simulink model "cvoo_g19_ponto4"  (R2021a)
settings: Solver=VariableStepAuto  StartTime=0.0  StopTime=100  RelTol=1e-3
values from neighbouring files (symbols this model uses):
  b_h_pt = [ ... (first row only)    [Ponto3.m]    (also in Ponto4.m; Ponto5.m)
  c_h_pt = eye(size(a_h_pt))    [Ponto3.m]    (also in Ponto4.m; Ponto5.m)
  conv_max = 5    [Ponto4.m]    (also in Ponto5.m)
  conv_min = 0    [Ponto4.m]    (also in Ponto5.m)
  conv_rms = 1.5*conv_res    (= 0.0018310546875)    [Ponto4.m]    (also in Ponto5.m)
  d_h_pt = zeros(size(b_h_pt))    [Ponto3.m]    (also in Ponto4.m; Ponto5.m)
  deg = pi/180    (= 0.0174532925199)    [Ponto2.m]    (also in Ponto3.m; Ponto4.m; Ponto5.m)
  f_amost = 100    [Ponto4.m]    (also in Ponto5.m)
  fat_conv_ra = 1/3    (= 0.333333333333)    [Ponto4.m]    (also in Ponto5.m)
  G_ra = 10e-3/ft    (= 0.0328083989501)    [Ponto4.m]    (also in Ponto5.m)
  G_sensq = (V_max_sensq-V_min_sensq)/(q_max_sensq-q_min_sensq)    (= 0.006)    [Ponto4.m]    (also in Ponto5.m)
  Gp_din = (v_pdin_max-v_pdin_min)/(pdin_max-pdin_min)    (= 0.00125)    [Ponto4.m]    (also in Ponto5.m)
  h_pt_ref = -1    [Ponto3.m]    (also in Ponto4.m; Ponto5.m = 0)
  h_ra_max = 1500*ft    (= 457.2)    [Ponto4.m]    (also in Ponto5.m)
  h_ra_min = 0    [Ponto4.m]    (also in Ponto5.m)
  K_lqr = lqr(a_h_pt_int, b_h_pt_int, Q, R)    [Ponto3.m]    (also in Ponto4.m; Ponto5.m)
  offset_alt = 150    [Ponto4.m]    (also in Ponto5.m = 0)
  offset_pdin = 2.5    [Ponto4.m]    (also in Ponto5.m)
  Offset_ra = 2.5    [Ponto4.m]    (also in Ponto5.m = 0)
  Offset_sensq = 2.5    [Ponto4.m]    (also in Ponto5.m)
  p_din_tau = 0.01    [Ponto4.m]    (also in Ponto5.m)
  pdin_max = 2e3    (= 2000)    [Ponto4.m]    (also in Ponto5.m)
  pdin_min = -2e3    (= -2000)    [Ponto4.m]    (also in Ponto5.m)
  q_max_sensq = 300    [Ponto4.m]    (also in Ponto5.m)
  q_min_sensq = -300    [Ponto4.m]    (also in Ponto5.m)
  ra_rms = 0.015    [Ponto4.m]    (also in Ponto5.m)
  rad = 180/pi    (= 57.2957795131)    [Ponto2.m]    (also in Ponto3.m; Ponto4.m; Ponto5.m)
  rho0 = 1.225    [Ponto4.m]    (also in Ponto5.m)
  rms_sensq = 4.4    [Ponto4.m]    (also in Ponto5.m)
  tau = 0.1    [Ponto4.m]    (also in Ponto5.m)
  u_ref = 0.4    [Ponto3.m]    (also in Ponto4.m; Ponto5.m = 0)
  vel_max_at = 60    [Ponto4.m]    (also in Ponto5.m)
  x0 = [0 0 0 0]    [Ponto3.m]    (also in Ponto4.m; Ponto5.m)
  x0_e = [0 0 0 0 0]    [Ponto4.m]    (also in Ponto5.m = [0 0 0 0 cond_ini.h0+h_solo_0])
undefined symbols (not defined in the file or in its folder): a_h_pt, ae, be, ce, cond_ini, de, max_deflec
libraries: simulink x5
settings Model: Creator=josem  LastModifiedBy=thomasmchilds
settings SolverCC: AlgebraicLoopSolver=TrustRegion
settings DebuggingCC: SFMachineParentedDataDiag=warning

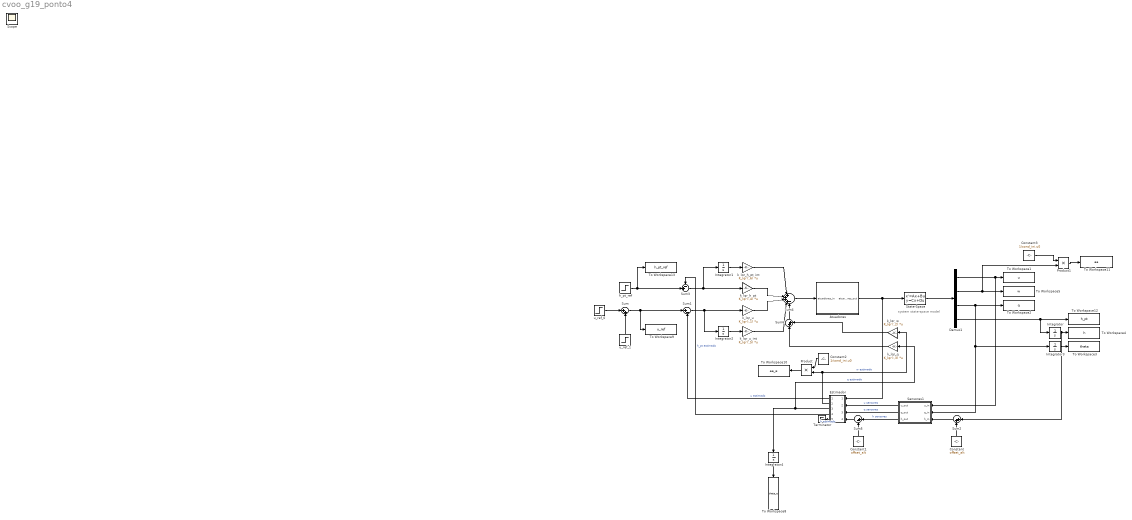
== system cvoo_g19_ponto4 ==
  note: system state-space model
  Atuadores : Subsystem
  Constant : Constant  Value=offset_alt
  Constant1 : Constant  Value=offset_alt
  Constant2 : Constant  Value=1/cond_ini.u0
  Constant3 : Constant  Value=1/cond_ini.u0
  Demux1 : Demux
  Estimador : Subsystem
  Integrator : Integrator
  Integrator1 : Integrator
  Integrator2 : Integrator
  Integrator3 : Integrator  InitialCondition=cond_ini.tt0
  Integrator4 : Integrator  InitialCondition=cond_ini.tt0
  Product : Product
  Product1 : Product
  Sensores1 : Subsystem
  State-Space : StateSpace  A=a_h_pt  B=b_h_pt  C=c_h_pt  D=d_h_pt  InitialCondition=x0
  Sum : Sum  Inputs=|++
  Sum1 : Sum  Inputs=|+-
  Sum2 : Sum  Inputs=|++
  Sum3 : Sum  Inputs=-+|
  Sum4 : Sum  Inputs=|++++-
  Sum5 : Sum  Inputs=|+-
  Sum6 : Sum  Inputs=|++
  Terminator : Terminator
  To Workspace1 : ToWorkspace  VariableName=u  SampleTime=-1
  To Workspace10 : ToWorkspace  VariableName=aa_e  SampleTime=-1
  To Workspace11 : ToWorkspace  VariableName=aa  SampleTime=-1
  To Workspace12 : ToWorkspace  VariableName=h_pt  SampleTime=-1
  To Workspace13 : ToWorkspace  VariableName=h_pt_ref  SampleTime=-1
  To Workspace2 : ToWorkspace  VariableName=q  SampleTime=-1
  To Workspace3 : ToWorkspace  VariableName=theta  SampleTime=-1
  To Workspace4 : ToWorkspace  VariableName=h  SampleTime=-1
  To Workspace5 : ToWorkspace  VariableName=w  SampleTime=-1
  To Workspace8 : ToWorkspace  VariableName=theta_e  SampleTime=-1
  To Workspace9 : ToWorkspace  VariableName=u_ref  SampleTime=-1
  h_pt_ref : Step  Time=50  After=h_pt_ref  SampleTime=0  VectorParams1D=off
  k_lqr_h_pt : Gain  Gain=K_lqr(:,4)  Multiplication=Matrix(K*u)
  k_lqr_h_pt_int : Gain  Gain=K_lqr(:,6)  Multiplication=Matrix(K*u)
  k_lqr_q : Gain  Gain=K_lqr(:,3)  Multiplication=Matrix(K*u)
  k_lqr_u : Gain  Gain=K_lqr(:,1)  Multiplication=Matrix(K*u)
  k_lqr_u_int : Gain  Gain=K_lqr(:,5)  Multiplication=Matrix(K*u)
  k_lqr_w : Gain  Gain=K_lqr(:,2)  Multiplication=Matrix(K*u)
  u_ref_0 : Step  Time=10  After=u_ref  SampleTime=0  VectorParams1D=off
  u_ref_1 : Step  Time=30  After=-u_ref  SampleTime=0
  Scope : Scope
  wires:
  h_pt_ref/1 -> Sum3/2, To Workspace13/1
  u_ref_0/1 -> Sum/1
  Integrator1/1 -> k_lqr_h_pt_int/1
  u_ref_1/1 -> Sum/2
  State-Space/1 -> Demux1/1
  k_lqr_u_int/1 -> Sum4/4
  Sum/1 -> To Workspace9/1, Sum1/1
  Sum1/1 -> Integrator2/1, k_lqr_u/1
  Demux1/3 -> To Workspace2/1, Sensores1/2(q_in), Integrator3/1
  Sum6/1 -> Sum4/5
  k_lqr_h_pt/1 -> Sum4/2
  Demux1/2 -> To Workspace5/1, Product1/2
  k_lqr_u/1 -> Sum4/3
  k_lqr_q/1 -> Sum6/1
  k_lqr_w/1 -> Sum6/2
  Sum4/1 -> Atuadores/1(atuadores_in)
  Demux1/4 -> Integrator/1, To Workspace12/1
  Atuadores/1(atuadores_out) -> State-Space/1, Estimador/1(In1)
  Sum3/1 -> Integrator1/1, k_lqr_h_pt/1
  Demux1/1 -> Sensores1/1(u_in), To Workspace1/1
  Integrator3/1 -> To Workspace3/1
  Integrator2/1 -> k_lqr_u_int/1
  Integrator/1 -> Sum2/1, To Workspace4/1
  k_lqr_h_pt_int/1 -> Sum4/1
  Sensores1/3(h_out) -> Sum5/1  "h sensores"
  Sensores1/2(q_out) -> Estimador/3(q_out)  "q sensores"
  Sum2/1 -> Sensores1/3(h_in)
  Constant/1 -> Sum2/2
  Constant1/1 -> Sum5/2
  Sum5/1 -> Estimador/4(h_out)
  Sensores1/1(u_out) -> Estimador/2(u_out)  "u sensores"
  Estimador/1(Out4) -> Sum1/2  "u estimado"
  Estimador/2(Out2) -> k_lqr_w/1, Product/2  "w estimado"
  Estimador/3(Out3) -> Integrator4/1, k_lqr_q/1  "q estimado"
  Estimador/4(Out1) -> Sum3/1  "h_pt estimado"
  Estimador/5(Out5) -> Terminator/1  "h estimado"
  Integrator4/1 -> To Workspace8/1
  Product/1 -> To Workspace10/1
  Constant2/1 -> Product/1
  Constant3/1 -> Product1/1
  Product1/1 -> To Workspace11/1

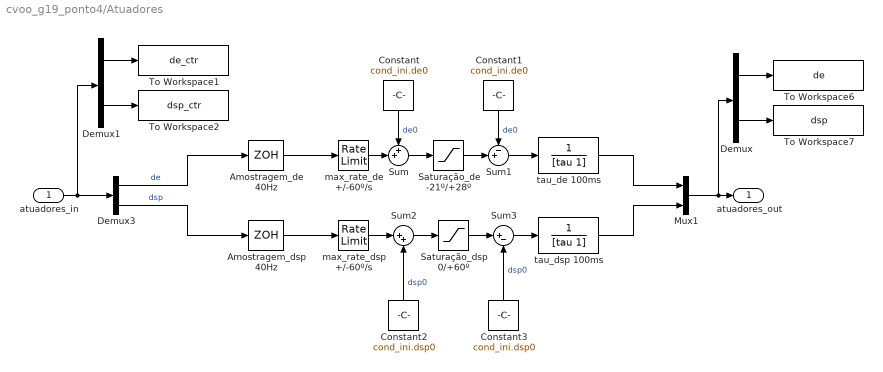
== system cvoo_g19_ponto4/Atuadores ==
  atuadores_in : Inport
  " max_rate_de +/-60º/s" : RateLimiter  RisingSlewLimit=vel_max_at*deg  FallingSlewLimit=-vel_max_at*deg  SampleTimeMode=inherited
  " max_rate_dsp +/-60º/s" : RateLimiter  RisingSlewLimit=vel_max_at*deg  FallingSlewLimit=-vel_max_at*deg  SampleTimeMode=inherited
  Amostragem_de 40Hz : ZeroOrderHold  SampleTime=1/f_amost
  Amostragem_dsp 40Hz : ZeroOrderHold  SampleTime=1/f_amost
  Constant : Constant  Value=cond_ini.de0
  Constant1 : Constant  Value=cond_ini.de0
  Constant2 : Constant  Value=cond_ini.dsp0
  Constant3 : Constant  Value=cond_ini.dsp0
  Demux : Demux  Outputs=2
  Demux1 : Demux  Outputs=2
  Demux3 : Demux  Outputs=2
  Mux1 : Mux  Inputs=2
  Saturação_de -21º/+28º : Saturate  UpperLimit=max_deflec.demax  LowerLimit=max_deflec.demin
  Saturação_dsp 0/+60º : Saturate  UpperLimit=max_deflec.spmax  LowerLimit=0
  Sum : Sum  Inputs=++|
  Sum1 : Sum  Inputs=-+|
  Sum2 : Sum  Inputs=|++
  Sum3 : Sum  Inputs=|+-
  To Workspace1 : ToWorkspace  VariableName=de_ctr  SaveFormat=Structure With Time  SampleTime=-1
  To Workspace2 : ToWorkspace  VariableName=dsp_ctr  SaveFormat=Structure With Time  SampleTime=-1
  To Workspace6 : ToWorkspace  VariableName=de  SaveFormat=Structure With Time  SampleTime=-1
  To Workspace7 : ToWorkspace  VariableName=dsp  SaveFormat=Structure With Time  SampleTime=-1
  tau_de 100ms : TransferFcn  Denominator=[tau 1]
  tau_dsp 100ms : TransferFcn  Denominator=[tau 1]
  atuadores_out : Outport
  wires:
  Mux1/1 -> Demux/1, atuadores_out/1
  atuadores_in/1 -> Demux1/1, Demux3/1
  Demux3/1 -> Amostragem_de 40Hz/1  "de"
  Demux3/2 -> Amostragem_dsp 40Hz/1  "dsp"
  tau_dsp 100ms/1 -> Mux1/2
  tau_de 100ms/1 -> Mux1/1
  Amostragem_dsp 40Hz/1 -> " max_rate_dsp +/-60º/s"/1
  Amostragem_de 40Hz/1 -> " max_rate_de +/-60º/s"/1
  " max_rate_de +/-60º/s"/1 -> Sum/2
  Sum/1 -> Saturação_de -21º/+28º/1
  Constant/1 -> Sum/1  "de0"
  Saturação_de -21º/+28º/1 -> Sum1/2
  Sum1/1 -> tau_de 100ms/1
  Constant1/1 -> Sum1/1  "de0"
  " max_rate_dsp +/-60º/s"/1 -> Sum2/1
  Sum2/1 -> Saturação_dsp 0/+60º/1
  Constant2/1 -> Sum2/2  "dsp0"
  Constant3/1 -> Sum3/2  "dsp0"
  Saturação_dsp 0/+60º/1 -> Sum3/1
  Sum3/1 -> tau_dsp 100ms/1
  Demux/1 -> To Workspace6/1
  Demux/2 -> To Workspace7/1
  Demux1/2 -> To Workspace2/1
  Demux1/1 -> To Workspace1/1

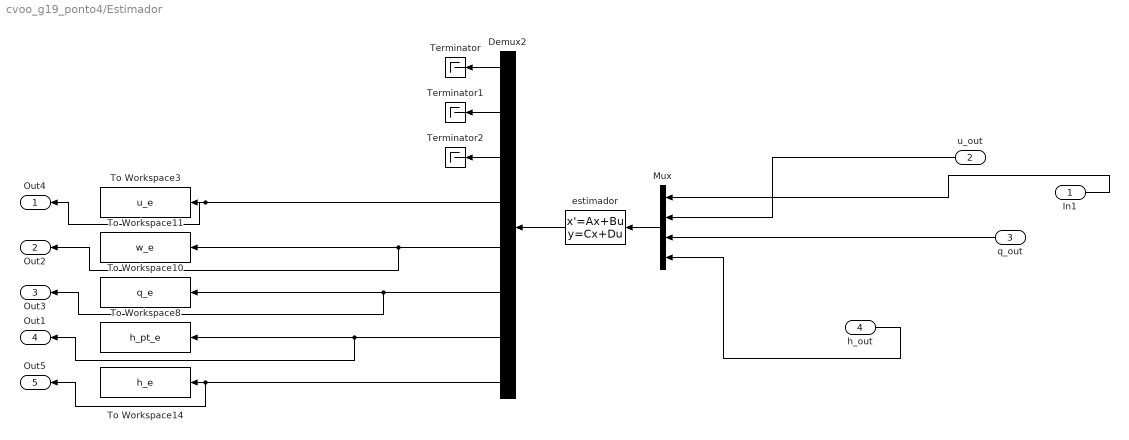
== system cvoo_g19_ponto4/Estimador ==
  In1 : Inport
  u_out : Inport  Port=2
  q_out : Inport  Port=3
  h_out : Inport  Port=4
  Demux2 : Demux  Outputs=8
  Mux : Mux
  Terminator : Terminator
  Terminator1 : Terminator
  Terminator2 : Terminator
  To Workspace10 : ToWorkspace  VariableName=q_e  SampleTime=-1
  To Workspace11 : ToWorkspace  VariableName=w_e  SampleTime=-1
  To Workspace14 : ToWorkspace  VariableName=h_e  SampleTime=-1
  To Workspace3 : ToWorkspace  VariableName=u_e  SampleTime=-1
  To Workspace8 : ToWorkspace  VariableName=h_pt_e  SampleTime=-1
  estimador : StateSpace  A=ae  B=be  C=ce  D=de  InitialCondition=x0_e
  Out4 : Outport
  Out2 : Outport  Port=2
  Out3 : Outport  Port=3
  Out1 : Outport  Port=4
  Out5 : Outport  Port=5
  wires:
  Demux2/2 -> Terminator1/1
  estimador/1 -> Demux2/1
  Demux2/5 -> Out2/1, To Workspace11/1
  Demux2/7 -> Out1/1, To Workspace8/1
  Demux2/8 -> Out5/1, To Workspace14/1
  Demux2/1 -> Terminator/1
  Demux2/4 -> Out4/1, To Workspace3/1
  Demux2/3 -> Terminator2/1
  Mux/1 -> estimador/1
  Demux2/6 -> Out3/1, To Workspace10/1
  In1/1 -> Mux/1
  q_out/1 -> Mux/3
  u_out/1 -> Mux/2
  h_out/1 -> Mux/4

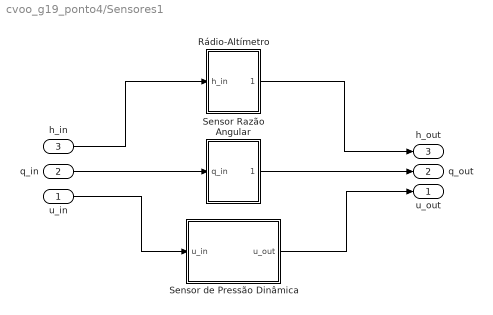
== system cvoo_g19_ponto4/Sensores1 ==
  u_in : Inport
  q_in : Inport  Port=2
  h_in : Inport  Port=3
  Rádio-Altímetro : Subsystem
  Sensor Razão Angular : Subsystem
  Sensor de Pressão Dinâmica : Subsystem
  u_out : Outport
  q_out : Outport  Port=2
  h_out : Outport  Port=3
  wires:
  Sensor Razão Angular/1(q_out) -> q_out/1
  u_in/1 -> Sensor de Pressão Dinâmica/1(u_in)
  Sensor de Pressão Dinâmica/1(u_out) -> u_out/1
  q_in/1 -> Sensor Razão Angular/1(q_in)
  h_in/1 -> Rádio-Altímetro/1(h_in)
  Rádio-Altímetro/1(h_out) -> h_out/1

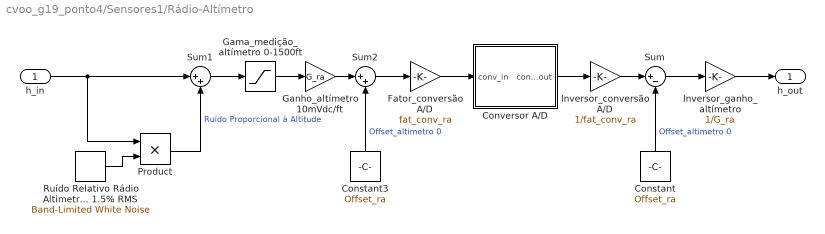
== system cvoo_g19_ponto4/Sensores1/Rádio-Altímetro ==
  h_in : Inport
  Constant : Constant  Value=Offset_ra
  Constant3 : Constant  Value=Offset_ra
  Conversor A/D : Subsystem
  Fator_conversão A/D : Gain  Gain=fat_conv_ra
  Gama_medição_altímetro 0-1500ft : Saturate  UpperLimit=h_ra_max  LowerLimit=h_ra_min
  Ganho_altímetro 10mVdc/ft : Gain  Gain=G_ra
  Inversor_conversão A/D : Gain  Gain=1/fat_conv_ra
  Inversor_ganho_altímetro : Gain  Gain=1/G_ra
  Product : Product
  Ruído Relativo Rádio Altimetro 1.5% RMS : simulink/Sources/Band-Limited White Noise  Cov=[ra_rms^2/f_amost]  Ts=1/f_amost  seed=[23341]
  Sum : Sum  Inputs=|+-
  Sum1 : Sum  Inputs=|++
  Sum2 : Sum  Inputs=|++
  h_out : Outport
  wires:
  Sum/1 -> Inversor_ganho_altímetro/1
  Constant/1 -> Sum/2  "Offset_altimetro 0"
  Sum2/1 -> Fator_conversão A/D/1
  Fator_conversão A/D/1 -> Conversor A/D/1(conv_in)
  Inversor_conversão A/D/1 -> Sum/1
  Conversor A/D/1(conv_out) -> Inversor_conversão A/D/1
  Inversor_ganho_altímetro/1 -> h_out/1
  h_in/1 -> Product/1, Sum1/1
  Sum1/1 -> Gama_medição_altímetro 0-1500ft/1
  Ganho_altímetro 10mVdc/ft/1 -> Sum2/1
  Gama_medição_altímetro 0-1500ft/1 -> Ganho_altímetro 10mVdc/ft/1
  Constant3/1 -> Sum2/2  "Offset_altimetro 0"
  Ruído Relativo Rádio Altimetro 1.5% RMS/1 -> Product/2
  Product/1 -> Sum1/2  "Ruído Proporcional à Altitude"

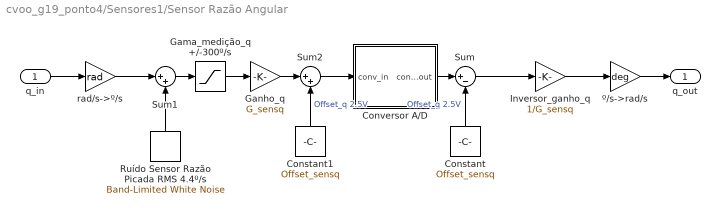
== system cvoo_g19_ponto4/Sensores1/Sensor Razão Angular ==
  q_in : Inport
  Constant : Constant  Value=Offset_sensq
  Constant1 : Constant  Value=Offset_sensq
  Conversor A/D : Subsystem
  Gama_medição_q +/-300º/s : Saturate  UpperLimit=q_max_sensq  LowerLimit=q_min_sensq
  Ganho_q : Gain  Gain=G_sensq
  Inversor_ganho_q : Gain  Gain=1/G_sensq
  Ruído Sensor Razão Picada RMS 4.4º/s : simulink/Sources/Band-Limited White Noise  Cov=[rms_sensq^2/f_amost]  Ts=1/f_amost  seed=[23341]
  Sum : Sum  Inputs=|+-
  Sum1 : Sum  Inputs=|++
  Sum2 : Sum  Inputs=|++
  rad/s->º/s : Gain  Gain=rad
  º/s->rad/s : Gain  Gain=deg
  q_out : Outport
  wires:
  Conversor A/D/1(conv_out) -> Sum/1
  Sum/1 -> Inversor_ganho_q/1
  Constant/1 -> Sum/2  "Offset_q 2.5V"
  Inversor_ganho_q/1 -> º/s->rad/s/1
  º/s->rad/s/1 -> q_out/1
  Sum1/1 -> Gama_medição_q +/-300º/s/1
  Gama_medição_q +/-300º/s/1 -> Ganho_q/1
  rad/s->º/s/1 -> Sum1/1
  Constant1/1 -> Sum2/2  "Offset_q 2.5V"
  Ganho_q/1 -> Sum2/1
  Ruído Sensor Razão Picada RMS 4.4º/s/1 -> Sum1/2
  q_in/1 -> rad/s->º/s/1
  Sum2/1 -> Conversor A/D/1(conv_in)

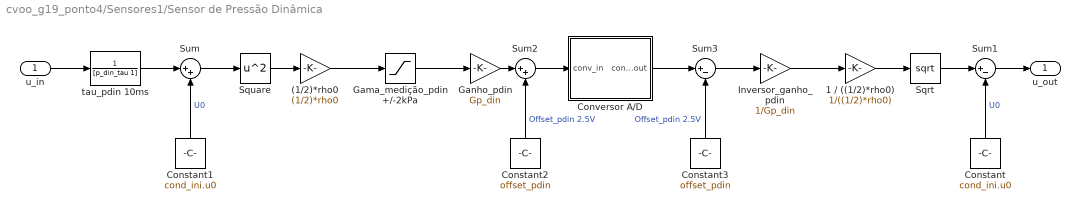
== system cvoo_g19_ponto4/Sensores1/Sensor de Pressão Dinâmica ==
  u_in : Inport
  (1/2)*rho0 : Gain  Gain=(1/2)*rho0
  1 / ((1/2)*rho0) : Gain  Gain=1/((1/2)*rho0)
  Constant : Constant  Value=cond_ini.u0
  Constant1 : Constant  Value=cond_ini.u0
  Constant2 : Constant  Value=offset_pdin
  Constant3 : Constant  Value=offset_pdin
  Conversor A/D : Subsystem
  Gama_medição_pdin +/-2kPa : Saturate  UpperLimit=pdin_max  LowerLimit=pdin_min
  Ganho_pdin : Gain  Gain=Gp_din
  Inversor_ganho_pdin : Gain  Gain=1/Gp_din
  Sqrt : Sqrt  SaturateOnIntegerOverflow=on
  Square : Math  Operator=square  SignedPower=on  SaturateOnIntegerOverflow=on
  Sum : Sum  Inputs=|++
  Sum1 : Sum  Inputs=|+-
  Sum2 : Sum  Inputs=|++
  Sum3 : Sum  Inputs=|+-
  tau_pdin 10ms : TransferFcn  Denominator=[p_din_tau 1]
  u_out : Outport
  wires:
  u_in/1 -> tau_pdin 10ms/1
  Sum/1 -> Square/1
  Ganho_pdin/1 -> Sum2/1
  Constant2/1 -> Sum2/2  "Offset_pdin 2.5V"
  tau_pdin 10ms/1 -> Sum/1
  (1/2)*rho0/1 -> Gama_medição_pdin +/-2kPa/1
  Constant1/1 -> Sum/2  "U0"
  Gama_medição_pdin +/-2kPa/1 -> Ganho_pdin/1
  Square/1 -> (1/2)*rho0/1
  Sum2/1 -> Conversor A/D/1(conv_in)
  Constant/1 -> Sum1/2  "U0"
  Sqrt/1 -> Sum1/1
  1 / ((1/2)*rho0)/1 -> Sqrt/1
  Inversor_ganho_pdin/1 -> 1 / ((1/2)*rho0)/1
  Sum3/1 -> Inversor_ganho_pdin/1
  Conversor A/D/1(conv_out) -> Sum3/1
  Sum1/1 -> u_out/1
  Constant3/1 -> Sum3/2  "Offset_pdin 2.5V"

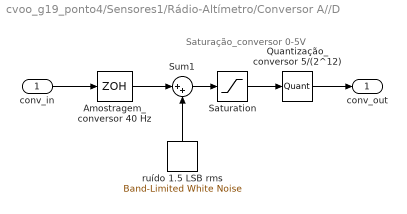
== system cvoo_g19_ponto4/Sensores1/Rádio-Altímetro/Conversor A//D ==
  note: Saturação_conversor
      |               0-5V
  conv_in : Inport
  Amostragem_conversor 40 Hz : ZeroOrderHold  SampleTime=1/f_amost
  Quantização_conversor 5/(2^12) : Quantizer  QuantizationInterval=fat_quant
  Saturation : Saturate  UpperLimit=conv_max  LowerLimit=conv_min
  Sum1 : Sum  Inputs=|++
  ruído 1.5 LSB rms : simulink/Sources/Band-Limited White Noise  Cov=[conv_rms^2/f_amost]  Ts=1/f_amost  seed=[23341]
  conv_out : Outport
  wires:
  conv_in/1 -> Amostragem_conversor 40 Hz/1
  Amostragem_conversor 40 Hz/1 -> Sum1/1
  ruído 1.5 LSB rms/1 -> Sum1/2
  Saturation/1 -> Quantização_conversor 5/(2^12)/1
  Sum1/1 -> Saturation/1
  Quantização_conversor 5/(2^12)/1 -> conv_out/1

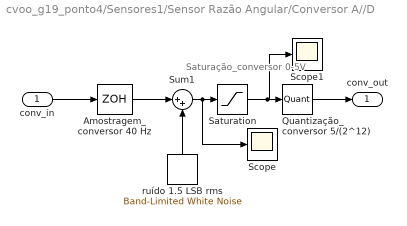
== system cvoo_g19_ponto4/Sensores1/Sensor Razão Angular/Conversor A//D ==
  note: Saturação_conversor
      |               0-5V
  conv_in : Inport
  Amostragem_conversor 40 Hz : ZeroOrderHold  SampleTime=1/f_amost
  Quantização_conversor 5/(2^12) : Quantizer  QuantizationInterval=fat_quant
  Saturation : Saturate  UpperLimit=conv_max  LowerLimit=conv_min
  Scope : Scope
  Scope1 : Scope
  Sum1 : Sum  Inputs=|++
  ruído 1.5 LSB rms : simulink/Sources/Band-Limited White Noise  Cov=[conv_rms^2/f_amost]  Ts=1/f_amost  seed=[23341]
  conv_out : Outport
  wires:
  conv_in/1 -> Amostragem_conversor 40 Hz/1
  Amostragem_conversor 40 Hz/1 -> Sum1/1
  ruído 1.5 LSB rms/1 -> Sum1/2
  Saturation/1 -> Scope1/1, Quantização_conversor 5/(2^12)/1
  Sum1/1 -> Scope/1, Saturation/1
  Quantização_conversor 5/(2^12)/1 -> conv_out/1

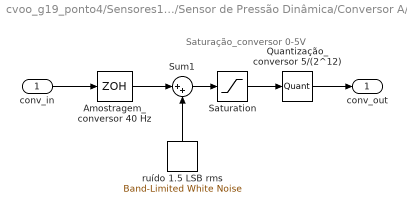
== system cvoo_g19_ponto4/Sensores1/Sensor de Pressão Dinâmica/Conversor A//D ==
  note: Saturação_conversor
      |               0-5V
  conv_in : Inport
  Amostragem_conversor 40 Hz : ZeroOrderHold  SampleTime=1/f_amost
  Quantização_conversor 5/(2^12) : Quantizer  QuantizationInterval=fat_quant
  Saturation : Saturate  UpperLimit=conv_max  LowerLimit=conv_min
  Sum1 : Sum  Inputs=|++
  ruído 1.5 LSB rms : simulink/Sources/Band-Limited White Noise  Cov=[conv_rms^2/f_amost]  Ts=1/f_amost  seed=[23341]
  conv_out : Outport
  wires:
  conv_in/1 -> Amostragem_conversor 40 Hz/1
  Amostragem_conversor 40 Hz/1 -> Sum1/1
  ruído 1.5 LSB rms/1 -> Sum1/2
  Saturation/1 -> Quantização_conversor 5/(2^12)/1
  Sum1/1 -> Saturation/1
  Quantização_conversor 5/(2^12)/1 -> conv_out/1
